simulink model "EXAMPLE_vrtkoff_hud"  (R2020a)
settings: Solver=ode45  StartTime=0.0  StopTime=15  RelTol=1e-3  EnableMultiTasking=on
libraries: vrlib x2, aerospace x1
Description:
  | Plane Take-Off with HUD Text
  | 
  | This model is a variant of the vrtkoff example that shows also how to display
  | signal values as text in the virtual scene and a simple Head-Up Display (HUD).
  | 
  | The text is sent to the virtual world as Simulink string signal, composed from the numeric
  | input values using the format string (see sprintf for more information) and sent
  | to the 'string' field of the corresponding Text node in the world. Individual lines of
  | the MFString field are separated by the newline character in the format string.
  | 
  | The HUD behavior (maintaining constant relative position between the user and the
  | Text node) is achieved by defining a ProximitySensor that senses user position and
  | orientation as it navigates through the scene and routing this information to the translation
  | and rotation of HUD object - in this case a VRML Transform that contains the Text node.
settings Model: EnablePacing=on  ExtModeTrigMode=oneshot  ExtModeArmWhenConnect=off  Creator=The MathWorks, Inc.  LastModifiedBy=augus
settings DataIOCC: LimitDataPoints=on  SaveFormat=Array  SaveOutput=off  SaveTime=off  ReturnWorkspaceOutputs=off  SignalLoggingName=logsOut
settings OptimizationCC: BlockReduction=off  BooleanDataType=off  ExpressionDepthLimit=2147483647  InitFltsAndDblsToZero=on  LifeSpan=inf
settings DebuggingCC: UnderspecifiedInitializationDetection=Classic  MergeDetectMultiDrivingBlocksExec=none  CheckExecutionContextPreStartOutputMsg=on  CheckExecutionContextRuntimeOutputMsg=on  SignalResolutionControl=TryResolveAllWithWarning  MultiTaskDSMMsg=warning  MultiTaskCondExecSysMsg=none  FcnCallInpInsideContextMsg=warning  StateNameClashWarn=warning  SymbolicDimsDataTypeCodeGenerationDiagnostic=none  SFUnexpectedBacktrackingDiag=warning  SFNoUnconditionalDefaultTransitionDiag=warning  SFExecutionAtInitializationDiag=none  ArithmeticOperatorsInVariantConditions=warning
settings HardwareCC: ProdBitPerPointer=32  ProdBitPerSizeT=32  ProdBitPerPtrDiffT=32  ProdLargestAtomicFloat=None  ProdIntDivRoundTo=Undefined  ProdEndianess=Unspecified  ProdWordSize=32  ProdHWDeviceType=32-bit Generic  TargetUnknown=on
settings ModelReferenceCC: UpdateModelReferenceTargets=IfOutOfDate  PropagateSignalLabelsOutOfModel=off
settings SFSimCC: SimUseLocalCustomCode=off  CustomCodeUndefinedFunction=UseInterfaceOnly
settings RTWCC: RTWUseLocalCustomCode=off
settings CodeAppCC: StateflowObjectComments=on
settings GRTTargetCC: TargetFcnLib=ansi_tfl_tmw.mat  TargetLangStandard=C89/C90 (ANSI)  CombineOutputUpdateFcns=off  GRTInterface=on
settings ConfigComp: CovMetricSettings=d  CovHtmlReporting=on  CovSaveCumulativeToWorkspaceVar=on  CovSaveSingleToWorkspaceVar=on  CovExternalEMLEnable=off  CovSFcnEnable=off

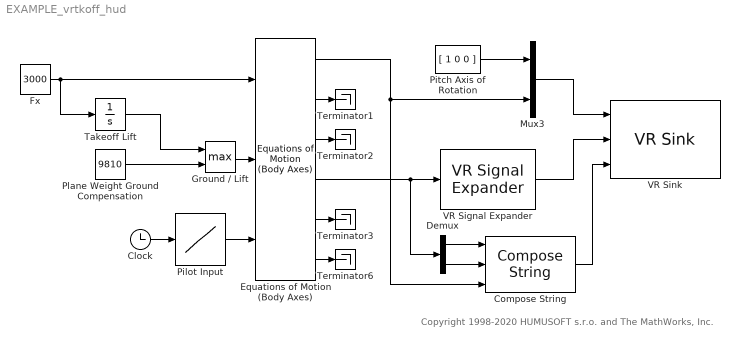
== system EXAMPLE_vrtkoff_hud ==
  note: Copyright 1998-2020 HUMUSOFT s.r.o. and The MathWorks, Inc.
  " Equations of Motion (Body Axes)" : aerospace/3DoF Equations of Motion / Equations of Motion (Body Axes)  v_ini=0  theta_ini=0  alpha_ini=0  q_ini=0  pos_ini=[0 0]  mass=1000  Iyy=1000  g=-9.81
      settings: SourceProductBaseCode=SL
  Clock : Clock
  Compose String : ComposeString  Format="'Xe      : %7.2f m\\nZe      : %7.2f m\\nAttitude: %7.2f rad'"
  Demux : Demux  Outputs=2
  Fx : Constant  Value=3000
  Ground / Lift : MinMax  Function=max  Inputs=2  InputSameDT=on  SaturateOnIntegerOverflow=on  ZeroCross=off
  Mux3 : Mux  Inputs=2
  Pilot Input : Lookup  InputValues=[0 1 2 8 9 15]  Table=[0 0 -20 20 0 0]  SaturateOnIntegerOverflow=on
  Pitch Axis of Rotation : Constant  Value=[ 1 0 0 ]
  Plane Weight Ground Compensation : Constant  Value=9810
  Takeoff Lift : Integrator  LimitOutput=on  UpperSaturationLimit=11000  LowerSaturationLimit=-Inf  ZeroCross=off
  Terminator{1..3,6} (4 alike) : Terminator
  VR Signal Expander : vrlib/VR Signal Expander  outwidth=3  outidx=[3 2]
  VR Sink : vrlib/VR Sink  InstantiateOnLoad=on  SampleTime=0.05  ViewEnable=on  RemoteChange=off  RemoteView=off  FieldsWritten=Plane.rotation.4.1.1.double#Plane.translation.3.1.1.double#HUDText1.string.1.-1.1.char  WorldFileName=vrtkoff_hud.x3d  WorldDescription=VR Plane Take-Off with HUD Text  AutoView=on  VideoDimensions=[]  AllowVariableSize=off
  wires:
  Pitch Axis of Rotation/1 -> Mux3/1
  " Equations of Motion (Body Axes)"/2 -> Terminator1/1
  " Equations of Motion (Body Axes)"/3 -> Terminator2/1
  Ground / Lift/1 -> " Equations of Motion (Body Axes)"/2
  Takeoff Lift/1 -> Ground / Lift/1
  Plane Weight Ground Compensation/1 -> Ground / Lift/2
  Clock/1 -> Pilot Input/1
  Pilot Input/1 -> " Equations of Motion (Body Axes)"/3
  Fx/1 -> " Equations of Motion (Body Axes)"/1, Takeoff Lift/1
  " Equations of Motion (Body Axes)"/6 -> Terminator6/1
  " Equations of Motion (Body Axes)"/5 -> Terminator3/1
  " Equations of Motion (Body Axes)"/1 -> Compose String/3, Mux3/2
  " Equations of Motion (Body Axes)"/4 -> Demux/1, VR Signal Expander/1
  Mux3/1 -> VR Sink/1
  VR Signal Expander/1 -> VR Sink/2
  Compose String/1 -> VR Sink/3
  Demux/1 -> Compose String/1
  Demux/2 -> Compose String/2
